simulink model "E55_1030"  (R2019b)
settings: Solver=FixedStepDiscrete  StartTime=0.0  StopTime=10  FixedStep=0.0005  RelTol=1e-3  EnableMultiTasking=on
InitFcn:
  | ecucoder_canfd
  | load('DATA_Plimit.mat')
  | a=0.775;
  | b=0.775;
  | kf=-50000;
  | kr=-50000;
  | m=226+75;
  | Iz=100;
  | u=0.85;
  | g=9.8;
  | L=a+b;
  | xi=0.1;
  | r=0.226;
  | Lw=1.171;
  | Tm=21;
  | i=15.9;
  | Jw=0.504;
  | Pmax=20000;
  | mw=19.3;
  | mb=148.9+75;
  | hg=0.280;
model workspace (MAT data in the model file):
  Initial_Steer_Position = 0
values from neighbouring files (symbols this model uses):
  SOC = [2.5 5 7.5 10 20 30 40 50 60 70 80 90 ... (14 elements, 14x1)]    [DATA_Plimit.mat]
  SOC_Discharge = [2.04592350211 2.57821618825 3.10671863859 3.63118835861 4.15200192786 4.66837694959 5.18149950051 5.69046162564 6.19532286188 6.696400261 7.19347596839 7.68712157998 ... (473 elements, 1x473)]    [DATA_Plimit.mat]
  VOLTAGE = [459.1488 476.0844 485.9448 487.344 492.822 498.8016 503.382 509.1108 518.8128 531.2472 544.5132 558.4656 ... (14 elements, 14x1)]    [DATA_Plimit.mat]
undefined symbols (not defined in the file or in its folder): DiscIntNeverNeededParam, H, HALL10, HALL6, HALL7, HALL8, HALL9, HPWM1, HPWM3, I_AN05_5V, I_AN07_5V, I_AN08_5V, I_AN09_5V, I_AN10_5V, I_SW11_H, I_SW12_H, I_SW13_H, I_SW14_H, I_SW15_H, I_SW16_H, I_SW17_H, I_SW18_H, I_SW19_H, LS1A2, O_HS1A2, O_HS1A8
libraries: ec311lib x152, simulink x92, canmsglib x30, canfdmsglib x2
(part 3 of 6)

== system E55_1030/Function-Call Subsystem3 ==
  CAN0 0X111 BMS CAN发送 : Inport
  function : TriggerPort  TriggerType=function-call  VariantControl=Variant
  Add : Sum
  Constant : Constant
  If : If  IfExpression=u1 >= 10
  If Action Subsystem : Subsystem  TreatAsAtomicUnit=on
  Saturation : Saturate  UpperLimit=10  LowerLimit=0
  Unit Delay : UnitDelay  SampleTime=-1  HasFrameUpgradeWarning=on
  wires:
  Unit Delay/1 -> Add/2
  Add/1 -> Saturation/1, Unit Delay/1
  Constant/1 -> Add/1
  CAN0 0X111 BMS CAN发送/1 -> If Action Subsystem/1(CAN0 0x111 BMS CAN发送)
  Saturation/1 -> If/1
  If/1 -> If Action Subsystem/Action

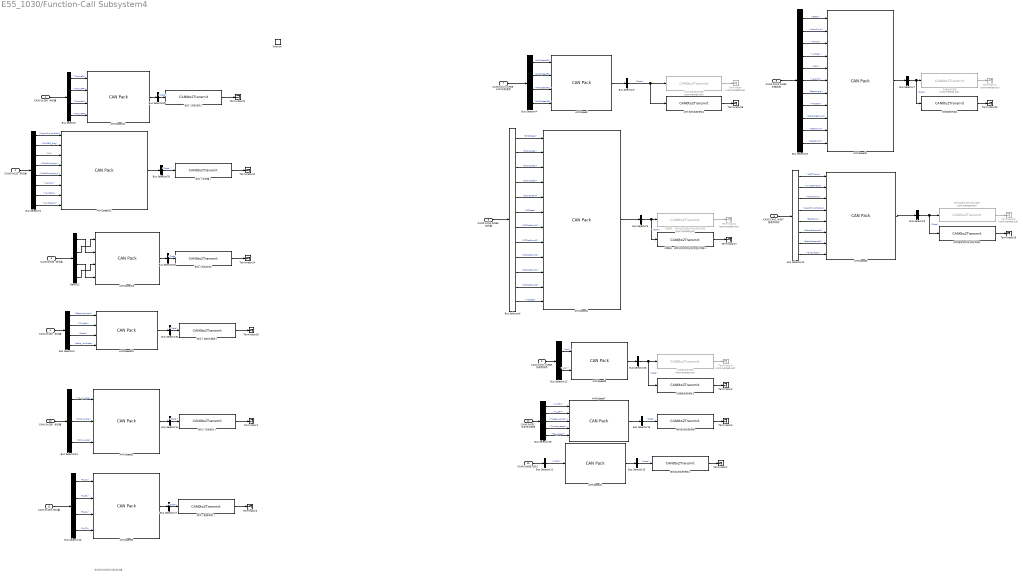
== system E55_1030/Function-Call Subsystem4 ==
  note: 驱动防滑和扭矩分配测试量
  CAN0 0x190 测试量 : Inport
  CAN0 0x191 测试量 : Inport  Port=2
  CAN0 0x192 测试量 : Inport  Port=3
  CAN0 0x194 测试量 : Inport  Port=4
  CAN0 CAN1 0x556 各种量 : Inport  Port=5
  CAN0 CAN1 0x557 温度和油压 : Inport  Port=6
  CAN0 CAN1 0x558 AMK电机速度 : Inport  Port=7
  CAN0 CAN1 0x559 车辆信息 : Inport  Port=8
  CAN0 CAN1 0x55B 加速度信息 : Inport  Port=9
  CAN0 0x195 测试量 : Inport  Port=10
  CAN0 0x193 测试量 : Inport  Port=11
  CAN0 0x55C 电机电流信息 : Inport  Port=12
  CAN0 0x55E vSOC : Inport  Port=13
  function : TriggerPort  TriggerType=function-call  VariantControl=Variant
  AMKSpeed : canmsglib/CAN Pack  MsgList=(none)  MsgName=AMKSpeed  MsgIDType=Standard (11-bit identifier)  MsgIdentifier=1368  MsgLength=8  Remote=off  ApplyMinMax=off  BusOutput=on  SignalInfo={ 'AMKSpeed1', '48', '16', 'LE', 'unsigned', 'Standard', '0', '1', '0', '0', '20000'; 'AMKSpeed2', '32', '16', 'LE', 'unsigned', 'Standard', '0', '1', '0', '0', '20000'; 'AMKSpeed3', '16', '16', 'LE', 'unsigned', 'Standard', '0', '1', '0', '0', '20000'; 'AMKSpeed4', '0', '16', 'LE', 'unsigned', 'Standard', '0', '1', '0', '0', '20000' }
      settings: SourceProductName=Vehicle Network Toolbox  SourceProductBaseCode=VN  DataFormat=manually specified signals
  AMKSpeed1 : canmsglib/CAN Pack  MsgList=(none)  MsgName=ErrorCode_State_Voltage  MsgIDType=Standard (11-bit identifier)  MsgIdentifier=1366  MsgLength=8  Remote=off  ApplyMinMax=off  BusOutput=on  SignalInfo={ 'BMS_State', '48', '1', 'LE', 'unsigned', 'Standard', '0', '1', '0', '0', '1'; 'Motor1_ErrorCode', '36', '12', 'LE', 'unsigned', 'Standard', '0', '1', '0', '0', '3871'; 'Motor2_ErrorCode', '24', '12', 'LE', 'unsigned', 'Standard', '0', '1', '0', '0', '3871'; 'Motor3_ErrorCode', '12', '12', 'LE', 'unsigned', 'Standard', '0', '1', '0', '0', '3871'; 'Motor4_ErrorCode', '0', '12', 'LE', 'unsigned', 'Standard', '0', '1', '0', '0', '3871'; 'SC_State', '49', '1', 'LE', 'unsigned', 'Standard', '0', '1', '0', '0', '1'; 'SC_TestPoint1', '50', '1', 'LE', 'unsigned', 'Standard', '0', '1', '0', '0', '1'; 'SC_TestPoint2', '51', '1', 'LE', 'unsigned', 'Standard', '0', '1', '0', '0', '1'; 'SC_TestPoint3', '52', '1', 'LE', 'unsigned', 'Standard', '0', '1', '0', '0', '1'; 'SC_TestPoint4', '53', '1', 'LE', 'unsigned', 'Standard', '0', '1', '0', '0', '1'; 'SC_TestPoint5', '54', '1', 'LE', 'unsigned', 'Standard', '0', '1', '0', '0', '1'; 'Voltage', '55', '9', 'LE', 'unsigned', 'Standard', '0', '0.1', '0', '0', '26' }
      settings: SourceProductName=Vehicle Network Toolbox  SourceProductBaseCode=VN  DataFormat=manually specified signals
  AMKSpeed11 : canmsglib/CAN Pack  MsgList=(none)  MsgName=Torque  MsgIDType=Standard (11-bit identifier)  MsgIdentifier=400  MsgLength=8  Remote=off  ApplyMinMax=off  BusOutput=on  SignalInfo={ 'TorqueFL', '16', '16', 'LE', 'signed', 'Standard', '0', '1', '0', '-Inf', 'Inf'; 'TorqueFR', '0', '16', 'LE', 'signed', 'Standard', '0', '1', '0', '-Inf', 'Inf'; 'TorqueRL', '48', '16', 'LE', 'signed', 'Standard', '0', '1', '0', '-Inf', 'Inf'; 'TorqueRR', '32', '16', 'LE', 'signed', 'Standard', '0', '1', '0', '-Inf', 'Inf' }
      settings: SourceProductName=Vehicle Network Toolbox  SourceProductBaseCode=VN  DataFormat=manually specified signals
  AMKSpeed12 : canmsglib/CAN Pack  MsgList=(none)  MsgName=Angle_Rate_Mz_Veloccity  MsgIDType=Standard (11-bit identifier)  MsgIdentifier=401  MsgLength=8  Remote=off  ApplyMinMax=off  BusOutput=on  SignalInfo={ 'Algorithm_Enable', '15', '1', 'LE', 'unsigned', 'Standard', '0', '1', '0', '0', '1'; 'K3105GStatus', '14', '1', 'LE', 'unsigned', 'Standard', '0', '1', '0', '0', '1'; 'Mz', '0', '14', 'LE', 'signed', 'Standard', '0', '0.05', '0', '-300', '300'; 'SideSlipAngle', '32', '8', 'LE', 'signed', 'Standard', '0', '0.1', '0', '-12.8', '12.7'; 'SideSlipAngle_d', '40', '8', 'LE', 'signed', 'Standard', '0', '0.1', '0', '-12.8', '12.7'; 'Velocity', '16', '16', 'LE', 'unsigned', 'Standard', '0', '0.01', '0', '0', '120'; 'YawRate', '48', '8', 'LE', 'signed', 'Standard', '0', '1', '0', '-128', '127'; 'YawRate_d', '56', '8', 'LE', 'signed', 'Standard', '0', '1', '0', '-128', '127' }
      settings: SourceProductName=Vehicle Network Toolbox  SourceProductBaseCode=VN  DataFormat=manually specified signals
  AMKSpeed13 : canmsglib/CAN Pack  MsgList=(none)  MsgName=Wheel_Speed  MsgIDType=Standard (11-bit identifier)  MsgIdentifier=402  MsgLength=8  Remote=off  ApplyMinMax=off  BusOutput=on  SignalInfo={ 'Wheel_Speed_FL', '0', '16', 'LE', 'signed', 'Standard', '0', '1', '0', '-1500', '1500'; 'Wheel_Speed_FR', '16', '16', 'LE', 'signed', 'Standard', '0', '1', '0', '-1500', '1500'; 'Wheel_Speed_RL', '32', '16', 'LE', 'signed', 'Standard', '0', '1', '0', '-1500', '1500'; 'Wheel_Speed_RR', '48', '16', 'LE', 'signed', 'Standard', '0', '1', '0', '-1500', '1500' }
      settings: SourceProductName=Vehicle Network Toolbox  SourceProductBaseCode=VN  DataFormat=manually specified signals
  AMKSpeed15 : canmsglib/CAN Pack  MsgList=(none)  MsgName=DriverIntention  MsgIDType=Standard (11-bit identifier)  MsgIdentifier=404  MsgLength=8  Remote=off  ApplyMinMax=off  BusOutput=on  SignalInfo={ 'SteeringAngle', '0', '12', 'LE', 'signed', 'Standard', '0', '0.01', '0', '-20', '20'; 'Throttle', '56', '8', 'LE', 'unsigned', 'Standard', '0', '1', '0', '0', '100'; 'break', '48', '8', 'LE', 'unsigned', 'Standard', '0', '1', '0', '0', '100'; 'delta_YawRate', '24', '8', 'LE', 'signed', 'Standard', '0', '1', '0', '-128', '127' }
      settings: SourceProductName=Vehicle Network Toolbox  SourceProductBaseCode=VN  DataFormat=manually specified signals
  AMKSpeed2 : canmsglib/CAN Pack  MsgList=(none)  MsgName=CarData  MsgIDType=Standard (11-bit identifier)  MsgIdentifier=1369  MsgLength=8  Remote=off  ApplyMinMax=off  BusOutput=on  SignalInfo={ 'Break', '51', '10', 'LE', 'unsigned', 'Standard', '0', '0.1', '0', '0', '100'; 'MotorAlive', '2', '4', 'LE', 'unsigned', 'Standard', '0', '1', '0', '0', '15'; 'Power', '17', '7', 'LE', 'signed', 'Standard', '0', '1', '44', '-20', '107'; 'RUN_Flag', '0', '2', 'LE', 'unsigned', 'Standard', '0', '1', '1', '1', '3'; 'SOC', '31', '10', 'LE', 'unsigned', 'Standard', '0', '0.1', '0', '0', '100'; 'Speed', '24', '7', 'LE', 'unsigned', 'Standard', '0', '1', '0', '0', '100'; 'SteerAngle', '6', '11', 'LE', 'signed', 'Standard', '0', '0.1', '0', '-100', '100'; 'Throttle', '41', '10', 'LE', 'unsigned', 'Standard', '0', '0.1', '0', '0', '100'; 'precharge_button', '63', '1', 'LE', 'unsigned', 'Standard', '0', '1', '0', '0', '1'; 'ready2go_button', '62', '1', 'LE', 'unsigned', 'Standard', '0', '1', '0', '0', '1'; 'reset_button', '61', '1', 'LE', 'unsigned', 'Standard', '0', '1', '0', '0', '1' }
      settings: SourceProductName=Vehicle Network Toolbox  SourceProductBaseCode=VN  DataFormat=manually specified signals
  AMKSpeed3 : canmsglib/CAN Pack  MsgList=(none)  MsgName=Temp_BreakPressure  MsgIDType=Standard (11-bit identifier)  MsgIdentifier=1367  MsgLength=8  Remote=off  ApplyMinMax=off  BusOutput=on  SignalInfo={ 'AMK_Temp_IGBT', '11', '11', 'LE', 'unsigned', 'Standard', '0', '0.1', '0', '0', '120'; 'AMK_Temp_Inverter', '22', '11', 'LE', 'unsigned', 'Standard', '0', '0.1', '0', '0', '120'; 'AMK_Temp_Motor', '33', '11', 'LE', 'unsigned', 'Standard', '0', '0.1', '0', '0', '120'; 'Algorithm_Enable', '63', '1', 'LE', 'unsigned', 'Standard', '0', '1', '0', '0', '1'; 'BattTemp', '0', '11', 'LE', 'unsigned', 'Standard', '0', '0.1', '0', '0', '120'; 'BreakPressure_F', '44', '9', 'LE', 'unsigned', 'Standard', '0', '0.05', '0', '0', '10'; 'BreakPressure_R', '53', '9', 'LE', 'unsigned', 'Standard', '0', '0.05', '0', '0', '10'; 'One_Motor', '62', '1', 'LE', 'unsigned', 'Standard', '0', '1', '0', '0', '1' }
      settings: SourceProductName=Vehicle Network Toolbox  SourceProductBaseCode=VN  DataFormat=manually specified signals
  AMKSpeed4 : canmsglib/CAN Pack  MsgList=(none)  MsgName=Dashboard_Control  MsgIDType=Standard (11-bit identifier)  MsgIdentifier=1374  MsgLength=8  Remote=off  ApplyMinMax=off  BusOutput=on  SignalInfo={ 'vSOC', '8', '16', 'LE', 'unsigned', 'Standard', '0', '0.01', '0', '0', '100' }
      settings: SourceProductName=Vehicle Network Toolbox  SourceProductBaseCode=VN  DataFormat=manually specified signals
  AMKSpeed5 : canmsglib/CAN Pack  MsgList=(none)  MsgName=Attitude  MsgIDType=Standard (11-bit identifier)  MsgIdentifier=405  MsgLength=8  Remote=off  ApplyMinMax=off  BusOutput=on  SignalInfo={ 'Heading_Angle', '0', '16', 'LE', 'unsigned', 'Standard', '0', '0.01', '0', '0', '360'; 'Pitch_Angle', '24', '16', 'LE', 'signed', 'Standard', '0', '0.01', '0', '-180', '180'; 'Roll_Angle', '48', '16', 'LE', 'signed', 'Standard', '0', '0.01', '0', '-180', '180' }
      settings: SourceProductName=Vehicle Network Toolbox  SourceProductBaseCode=VN  DataFormat=manually specified signals
  AMKSpeed6 : canmsglib/CAN Pack  MsgList=(none)  MsgName=Fz  MsgIDType=Standard (11-bit identifier)  MsgIdentifier=403  MsgLength=8  Remote=off  ApplyMinMax=off  BusOutput=on  SignalInfo={ 'Fz_FL', '0', '16', 'LE', 'unsigned', 'Standard', '0', '0.05', '0', '0', '2000'; 'Fz_FR', '16', '16', 'LE', 'unsigned', 'Standard', '0', '0.05', '0', '0', '2000'; 'Fz_RL', '32', '16', 'LE', 'unsigned', 'Standard', '0', '0.05', '0', '0', '2000'; 'Fz_RR', '48', '16', 'LE', 'unsigned', 'Standard', '0', '0.05', '0', '0', '2000' }
      settings: SourceProductName=Vehicle Network Toolbox  SourceProductBaseCode=VN  DataFormat=manually specified signals
  AMKSpeed7 : canmsglib/CAN Pack  MsgList=(none)  MsgName=Current  MsgIDType=Standard (11-bit identifier)  MsgIdentifier=1372  MsgLength=8  Remote=off  ApplyMinMax=off  BusOutput=on  SignalInfo={ 'Id_284', '0', '16', 'LE', 'signed', 'Standard', '0', '0.001', '0', '-10', '20'; 'Iq_284', '16', '16', 'LE', 'signed', 'Standard', '0', '0.001', '0', '-10', '20'; 'Target_velocity', '32', '16', 'LE', 'signed', 'Standard', '0', '1', '0', '-5000', '20000'; 'Torque_regen', '49', '15', 'LE', 'signed', 'Standard', '0', '0.1', '0', '-1000', '0'; 'flag_regen', '48', '1', 'LE', 'unsigned', 'Standard', '0', '1', '0', '0', '1' }
      settings: SourceProductName=Vehicle Network Toolbox  SourceProductBaseCode=VN  DataFormat=manually specified signals
  AMKSpeed9 : canmsglib/CAN Pack  MsgList=(none)  MsgName=Acceleration  MsgIDType=Standard (11-bit identifier)  MsgIdentifier=1371  MsgLength=8  Remote=off  ApplyMinMax=off  BusOutput=on  SignalInfo={ 'Acceleration_X', '0', '16', 'LE', 'signed', 'Standard', '0', '0.01', '0', '-40', '40'; 'Acceleration_Y', '16', '16', 'LE', 'signed', 'Standard', '0', '0.01', '0', '-40', '40' }
      settings: SourceProductName=Vehicle Network Toolbox  SourceProductBaseCode=VN  DataFormat=manually specified signals
  AMK电机速度传输 : ec311lib/RapidECU_U34/03CANCommunication/CAN0to2Transmit  Commented=on  canmodule=1  canbuffer=29  canmessageid=hex2dec('0558')  canmessagetype=Standard(11-bit ID)  datalength=8  sampletime=-1
      settings: SourceProductName=ECUCoder for S32K311
  AMK电机速度传输1 : ec311lib/RapidECU_U34/03CANCommunication/CAN0to2Transmit  canmodule=0  canbuffer=29  canmessageid=hex2dec('0558')  canmessagetype=Standard(11-bit ID)  datalength=8  sampletime=-1
      settings: SourceProductName=ECUCoder for S32K311
  Bus Selector : BusSelector  OutputSignals=TorqueFL,TorqueFR,TorqueRL,TorqueRR
  Bus Selector1 : BusSelector  OutputSignals=Algorithm_Enable,K3105G_flag,Mz,SideSlipAngle,SideSlipAngle_d,velocity,YawRate,YawRate_d
  Bus Selector10 : BusSelector  OutputSignals=IGBTTemp,InverterTemp,MotorTemp,Algorithm_Enable,BattTemp,BreakPressureF,BreakPressureR,One_Motor
  Bus Selector11 : BusSelector  OutputSignals=vSOC
  Bus Selector12 : BusSelector  OutputSignals=AccX,AccY
  Bus Selector13 : BusSelector  OutputSignals=Yaw_Angle,Pitch_Angle,Roll_Angle
  Bus Selector{3,5,7,9,14..15,17..18,26,28..30,32} (13 alike) : BusSelector  OutputSignals=Data
  Bus Selector16 : BusSelector  OutputSignals=Fz_FL,Fz_FR,Fz_RL,Fz_RR
  Bus Selector19 : BusSelector  OutputSignals=Id_284,Iq_284,Target_velocity,Torque_regen,flag_regen
  Bus Selector2 : BusSelector  OutputSignals=SteeringAngle,Throttle,Break,delta_YawRate
  Bus Selector4 : BusSelector  OutputSignals=AMKSpeedFL,AMKSpeedFR,AMKSpeedRL,AMKSpeedRR
  Bus Selector6 : BusSelector  OutputSignals=BMSState,ErrorCode1,ErrorCode2,ErrorCode3,ErrorCode4,SCState,SCTestPoint1,SCTestPoint2,SCTestPoint3,SCTestPoint4,SCTestPoint5,Voltage
  Bus Selector8 : BusSelector  OutputSignals=Break,MotorAlive,Power,runflag,SOC,velocity,SteerAngle,Throttle,PrechargeInput,StartInput,ResetInput
  Demux2 : Demux
  Terminator{,4,7..9} (5 alike) : Terminator  Commented=on
  Terminator{1..3,5..6,22,24..28,30..31} (13 alike) : Terminator
  加速度信息传输 : ec311lib/RapidECU_U34/03CANCommunication/CAN0to2Transmit  Commented=on  canmodule=1  canbuffer=1  canmessageid=hex2dec('055B')  canmessagetype=Standard(11-bit ID)  datalength=8  sampletime=-1
      settings: SourceProductName=ECUCoder for S32K311
  加速度信息传输1 : ec311lib/RapidECU_U34/03CANCommunication/CAN0to2Transmit  canmodule=0  canbuffer=1  canmessageid=hex2dec('055B')  canmessagetype=Standard(11-bit ID)  datalength=8  sampletime=-1
      settings: SourceProductName=ECUCoder for S32K311
  各种温度和刹车油压传输 : ec311lib/RapidECU_U34/03CANCommunication/CAN0to2Transmit  Commented=on  canmodule=1  canbuffer=31  canmessageid=hex2dec('0557')  canmessagetype=Standard(11-bit ID)  datalength=8  sampletime=-1
      settings: SourceProductName=ECUCoder for S32K311
  各种温度和刹车油压传输1 : ec311lib/RapidECU_U34/03CANCommunication/CAN0to2Transmit  canmodule=0  canbuffer=31  canmessageid=hex2dec('0557')  canmessagetype=Standard(11-bit ID)  datalength=8  sampletime=-1
      settings: SourceProductName=ECUCoder for S32K311
  故障码、各种状态和低压电池电压传输 : ec311lib/RapidECU_U34/03CANCommunication/CAN0to2Transmit  Commented=on  canmodule=1  canbuffer=30  canmessageid=hex2dec('0556')  canmessagetype=Standard(11-bit ID)  datalength=8  sampletime=-1
      settings: SourceProductName=ECUCoder for S32K311
  故障码、各种状态和低压电池电压传输1 : ec311lib/RapidECU_U34/03CANCommunication/CAN0to2Transmit  canmodule=0  canbuffer=30  canmessageid=hex2dec('0556')  canmessagetype=Standard(11-bit ID)  datalength=8  sampletime=-1
      settings: SourceProductName=ECUCoder for S32K311
  测试（各种量） : ec311lib/RapidECU_U34/03CANCommunication/CAN0to2Transmit  canmodule=0  canbuffer=13  canmessageid=hex2dec('0191')  canmessagetype=Standard(11-bit ID)  datalength=8  sampletime=-1
      settings: SourceProductName=ECUCoder for S32K311
  测试（四轮扭矩） : ec311lib/RapidECU_U34/03CANCommunication/CAN0to2Transmit  canmodule=0  canbuffer=12  canmessageid=hex2dec('0190')  canmessagetype=Standard(11-bit ID)  datalength=8  sampletime=-1
      settings: SourceProductName=ECUCoder for S32K311
  测试（四轮轮速） : ec311lib/RapidECU_U34/03CANCommunication/CAN0to2Transmit  canmodule=0  canbuffer=14  canmessageid=hex2dec('0192')  canmessagetype=Standard(11-bit ID)  datalength=8  sampletime=-1
      settings: SourceProductName=ECUCoder for S32K311
  测试（垂直载荷） : ec311lib/RapidECU_U34/03CANCommunication/CAN0to2Transmit  canmodule=0  canbuffer=17  canmessageid=hex2dec('0193')  canmessagetype=Standard(11-bit ID)  datalength=8  sampletime=-1
      settings: SourceProductName=ECUCoder for S32K311
  测试（车身姿态） : ec311lib/RapidECU_U34/03CANCommunication/CAN0to2Transmit  canmodule=0  canbuffer=18  canmessageid=hex2dec('0195')  canmessagetype=Standard(11-bit ID)  datalength=8  sampletime=-1
      settings: SourceProductName=ECUCoder for S32K311
  测试（驾驶员意图） : ec311lib/RapidECU_U34/03CANCommunication/CAN0to2Transmit  canmodule=0  canbuffer=16  canmessageid=hex2dec('0194')  canmessagetype=Standard(11-bit ID)  datalength=8  sampletime=-1
      settings: SourceProductName=ECUCoder for S32K311
  电机电流信息传输 : ec311lib/RapidECU_U34/03CANCommunication/CAN0to2Transmit  canmodule=0  canbuffer=33  canmessageid=hex2dec('055C')  canmessagetype=Standard(11-bit ID)  datalength=8  sampletime=-1
      settings: SourceProductName=ECUCoder for S32K311
  电机电流信息传输1 : ec311lib/RapidECU_U34/03CANCommunication/CAN0to2Transmit  canmodule=0  canbuffer=34  canmessageid=hex2dec('055E')  canmessagetype=Standard(11-bit ID)  datalength=8  sampletime=-1
      settings: SourceProductName=ECUCoder for S32K311
  车辆信息传输 : ec311lib/RapidECU_U34/03CANCommunication/CAN0to2Transmit  Commented=on  canmodule=1  canbuffer=32  canmessageid=hex2dec('0559')  canmessagetype=Standard(11-bit ID)  datalength=8  sampletime=-1
      settings: SourceProductName=ECUCoder for S32K311
  车辆信息传输1 : ec311lib/RapidECU_U34/03CANCommunication/CAN0to2Transmit  canmodule=0  canbuffer=32  canmessageid=hex2dec('0559')  canmessagetype=Standard(11-bit ID)  datalength=8  sampletime=-1
      settings: SourceProductName=ECUCoder for S32K311
  wires:
  测试（四轮扭矩）/1 -> Terminator31/1
  测试（驾驶员意图）/1 -> Terminator30/1
  测试（各种量）/1 -> Terminator22/1
  测试（四轮轮速）/1 -> Terminator24/1
  车辆信息传输1/1 -> Terminator25/1
  各种温度和刹车油压传输1/1 -> Terminator26/1
  各种温度和刹车油压传输/1 -> Terminator8/1
  车辆信息传输/1 -> Terminator7/1
  故障码、各种状态和低压电池电压传输/1 -> Terminator4/1
  故障码、各种状态和低压电池电压传输1/1 -> Terminator27/1
  AMK电机速度传输/1 -> Terminator/1
  AMK电机速度传输1/1 -> Terminator28/1
  加速度信息传输/1 -> Terminator9/1
  AMKSpeed11/1 -> Bus Selector29/1
  Bus Selector29/1 -> 测试（四轮扭矩）/1  "<Data>"
  CAN0 0x190 测试量/1 -> Bus Selector/1
  Bus Selector/1 -> AMKSpeed11/1  "<TorqueFL>"
  Bus Selector/2 -> AMKSpeed11/2  "<TorqueFR>"
  Bus Selector/3 -> AMKSpeed11/3  "<TorqueRL>"
  Bus Selector/4 -> AMKSpeed11/4  "<TorqueRR>"
  AMKSpeed12/1 -> Bus Selector28/1
  Bus Selector28/1 -> 测试（各种量）/1  "<Data>"
  CAN0 0x191 测试量/1 -> Bus Selector1/1
  Demux2/1 -> AMKSpeed13/2
  Demux2/3 -> AMKSpeed13/4
  Demux2/2 -> AMKSpeed13/1
  Demux2/4 -> AMKSpeed13/3
  AMKSpeed13/1 -> Bus Selector30/1
  CAN0 0x192 测试量/1 -> Demux2/1
  Bus Selector30/1 -> 测试（四轮轮速）/1  "<Data>"
  AMKSpeed15/1 -> Bus Selector32/1
  Bus Selector32/1 -> 测试（驾驶员意图）/1  "<Data>"
  CAN0 0x194 测试量/1 -> Bus Selector2/1
  AMKSpeed/1 -> Bus Selector3/1
  CAN0 CAN1 0x558 AMK电机速度/1 -> Bus Selector4/1
  Bus Selector4/1 -> AMKSpeed/1  "<AMKSpeedFL>"
  Bus Selector4/2 -> AMKSpeed/2  "<AMKSpeedFR>"
  Bus Selector4/3 -> AMKSpeed/3  "<AMKSpeedRL>"
  Bus Selector4/4 -> AMKSpeed/4  "<AMKSpeedRR>"
  Bus Selector3/1 -> AMK电机速度传输1/1, AMK电机速度传输/1  "<Data>"
  AMKSpeed1/1 -> Bus Selector5/1
  Bus Selector5/1 -> 故障码、各种状态和低压电池电压传输1/1, 故障码、各种状态和低压电池电压传输/1  "<Data>"
  CAN0 CAN1 0x556 各种量/1 -> Bus Selector6/1
  Bus Selector6/1 -> AMKSpeed1/1  "<BMSState>"
  Bus Selector6/2 -> AMKSpeed1/2  "<ErrorCode1>"
  Bus Selector6/3 -> AMKSpeed1/3  "<ErrorCode2>"
  Bus Selector6/4 -> AMKSpeed1/4  "<ErrorCode3>"
  Bus Selector6/5 -> AMKSpeed1/5  "<ErrorCode4>"
  Bus Selector6/6 -> AMKSpeed1/6  "<SCState>"
  Bus Selector6/7 -> AMKSpeed1/7  "<SCTestPoint1>"
  Bus Selector6/8 -> AMKSpeed1/8  "<SCTestPoint2>"
  Bus Selector6/9 -> AMKSpeed1/9  "<SCTestPoint3>"
  Bus Selector6/10 -> AMKSpeed1/10  "<SCTestPoint4>"
  Bus Selector6/11 -> AMKSpeed1/11  "<SCTestPoint5>"
  Bus Selector6/12 -> AMKSpeed1/12  "<Voltage>"
  AMKSpeed2/1 -> Bus Selector7/1
  Bus Selector7/1 -> 车辆信息传输1/1, 车辆信息传输/1  "<Data>"
  CAN0 CAN1 0x559 车辆信息/1 -> Bus Selector8/1
  Bus Selector8/1 -> AMKSpeed2/1  "<Break>"
  Bus Selector8/2 -> AMKSpeed2/2  "<MotorAlive>"
  Bus Selector8/3 -> AMKSpeed2/3  "<Power>"
  Bus Selector8/4 -> AMKSpeed2/4  "<runflag>"
  Bus Selector8/5 -> AMKSpeed2/5  "<SOC>"
  Bus Selector8/6 -> AMKSpeed2/6  "<velocity>"
  Bus Selector8/7 -> AMKSpeed2/7  "<SteerAngle>"
  Bus Selector8/8 -> AMKSpeed2/8  "<Throttle>"
  Bus Selector8/9 -> AMKSpeed2/9  "<PrechargeInput>"
  Bus Selector8/10 -> AMKSpeed2/10  "<StartInput>"
  Bus Selector8/11 -> AMKSpeed2/11  "<ResetInput>"
  AMKSpeed3/1 -> Bus Selector9/1
  Bus Selector9/1 -> 各种温度和刹车油压传输1/1, 各种温度和刹车油压传输/1  "<Data>"
  CAN0 CAN1 0x557 温度和油压/1 -> Bus Selector10/1
  Bus Selector10/1 -> AMKSpeed3/1  "<IGBTTemp>"
  Bus Selector10/2 -> AMKSpeed3/2  "<InverterTemp>"
  Bus Selector10/3 -> AMKSpeed3/3  "<MotorTemp>"
  AMKSpeed9/1 -> Bus Selector26/1
  Bus Selector26/1 -> 加速度信息传输1/1, 加速度信息传输/1  "<Data>"
  CAN0 CAN1 0x55B 加速度信息/1 -> Bus Selector12/1
  Bus Selector12/1 -> AMKSpeed9/1  "<AccX>"
  Bus Selector12/2 -> AMKSpeed9/2  "<AccY>"
  Bus Selector10/5 -> AMKSpeed3/5  "<BattTemp>"
  Bus Selector10/6 -> AMKSpeed3/6  "<BreakPressureF>"
  Bus Selector10/7 -> AMKSpeed3/7  "<BreakPressureR>"
  Bus Selector10/4 -> AMKSpeed3/4  "<Algorithm_Enable>"
  Bus Selector1/1 -> AMKSpeed12/1  "<Algorithm_Enable>"
  Bus Selector1/2 -> AMKSpeed12/2  "<K3105G_flag>"
  Bus Selector1/3 -> AMKSpeed12/3  "<Mz>"
  Bus Selector1/4 -> AMKSpeed12/4  "<SideSlipAngle>"
  Bus Selector1/5 -> AMKSpeed12/5  "<SideSlipAngle_d>"
  Bus Selector1/6 -> AMKSpeed12/6  "<velocity>"
  Bus Selector1/7 -> AMKSpeed12/7  "<YawRate>"
  Bus Selector1/8 -> AMKSpeed12/8  "<YawRate_d>"
  Bus Selector14/1 -> 测试（车身姿态）/1  "<Data>"
  CAN0 0x195 测试量/1 -> Bus Selector13/1
  测试（车身姿态）/1 -> Terminator1/1
  AMKSpeed5/1 -> Bus Selector14/1
  Bus Selector13/1 -> AMKSpeed5/1  "<Yaw_Angle>"
  Bus Selector13/2 -> AMKSpeed5/2  "<Pitch_Angle>"
  Bus Selector13/3 -> AMKSpeed5/3  "<Roll_Angle>"
  加速度信息传输1/1 -> Terminator3/1
  Bus Selector2/1 -> AMKSpeed15/1  "<SteeringAngle>"
  Bus Selector2/2 -> AMKSpeed15/2  "<Throttle>"
  Bus Selector2/3 -> AMKSpeed15/3  "<Break>"
  Bus Selector10/8 -> AMKSpeed3/8  "<One_Motor>"
  Bus Selector2/4 -> AMKSpeed15/4  "<delta_YawRate>"
  AMKSpeed6/1 -> Bus Selector17/1
  测试（垂直载荷）/1 -> Terminator5/1
  Bus Selector17/1 -> 测试（垂直载荷）/1  "<Data>"
  CAN0 0x193 测试量/1 -> Bus Selector16/1
  Bus Selector16/4 -> AMKSpeed6/4  "<Fz_RR>"
  Bus Selector16/3 -> AMKSpeed6/3  "<Fz_RL>"
  Bus Selector16/2 -> AMKSpeed6/2  "<Fz_FR>"
  Bus Selector16/1 -> AMKSpeed6/1  "<Fz_FL>"
  AMKSpeed7/1 -> Bus Selector18/1
  Bus Selector18/1 -> 电机电流信息传输/1  "<Data>"
  电机电流信息传输/1 -> Terminator6/1
  CAN0 0x55C 电机电流信息/1 -> Bus Selector19/1
  Bus Selector19/1 -> AMKSpeed7/1  "<Id_284>"
  Bus Selector19/2 -> AMKSpeed7/2  "<Iq_284>"
  Bus Selector19/4 -> AMKSpeed7/4  "<Torque_regen>"
  Bus Selector19/5 -> AMKSpeed7/5  "<flag_regen>"
  Bus Selector19/3 -> AMKSpeed7/3  "<Target_velocity>"
  CAN0 0x55E vSOC/1 -> Bus Selector11/1
  Bus Selector11/1 -> AMKSpeed4/1  "<vSOC>"
  电机电流信息传输1/1 -> Terminator2/1
  Bus Selector15/1 -> 电机电流信息传输1/1  "<Data>"
  AMKSpeed4/1 -> Bus Selector15/1

== system E55_1030/Function-Call Subsystem5 ==
  CAN2 0x185 右前 : Inport
  CAN2 0x184 左前 : Inport  Port=2
  CAN2 0x189 右后 : Inport  Port=3
  CAN2 0x188 左后 : Inport  Port=4
  function : TriggerPort  TriggerType=function-call  VariantControl=Variant
  AMKSpeed5 : canmsglib/CAN Pack  MsgList=(none)  MsgName=VCU4_0x184  MsgIDType=Standard (11-bit identifier)  MsgIdentifier=388  MsgLength=8  Remote=off  ApplyMinMax=off  BusOutput=on  SignalInfo={ 'DcOn', '9', '1', 'LE', 'unsigned', 'Standard', '0', '1', '0', '0', '1'; 'Enable', '10', '1', 'LE', 'unsigned', 'Standard', '0', '1', '0', '0', '1'; 'ErrorReset', '11', '1', 'LE', 'unsigned', 'Standard', '0', '1', '0', '0', '1'; 'InverterOn', '8', '1', 'LE', 'unsigned', 'Standard', '0', '1', '0', '-Inf', 'Inf'; 'TargetVelocity', '16', '16', 'LE', 'signed', 'Standard', '0', '1', '0', '-32768', '32767'; 'TorqueLimitNegativ', '48', '16', 'LE', 'signed', 'Standard', '0', '1', '0', '-32768', '32767'; 'TorqueLimitPositiv', '32', '16', 'LE', 'signed', 'Standard', '0', '1', '0', '-32768', '32767' }
      settings: SourceProductName=Vehicle Network Toolbox  SourceProductBaseCode=VN  DataFormat=manually specified signals
  AMKSpeed6 : canmsglib/CAN Pack  MsgList=(none)  MsgName=VCU4_0x185  MsgIDType=Standard (11-bit identifier)  MsgIdentifier=389  MsgLength=8  Remote=off  ApplyMinMax=off  BusOutput=on  SignalInfo={ 'DcOn', '9', '1', 'LE', 'unsigned', 'Standard', '0', '1', '0', '0', '1'; 'Enable', '10', '1', 'LE', 'unsigned', 'Standard', '0', '1', '0', '0', '1'; 'ErrorReset', '11', '1', 'LE', 'unsigned', 'Standard', '0', '1', '0', '0', '1'; 'InverterOn', '8', '1', 'LE', 'unsigned', 'Standard', '0', '1', '0', '-Inf', 'Inf'; 'TargetVelocity', '16', '16', 'LE', 'signed', 'Standard', '0', '1', '0', '-32768', '32767'; 'TorqueLimitNegativ', '48', '16', 'LE', 'signed', 'Standard', '0', '1', '0', '-32768', '32767'; 'TorqueLimitPositiv', '32', '16', 'LE', 'signed', 'Standard', '0', '1', '0', '-32768', '32767' }
      settings: SourceProductName=Vehicle Network Toolbox  SourceProductBaseCode=VN  DataFormat=manually specified signals
  AMKSpeed7 : canmsglib/CAN Pack  MsgList=(none)  MsgName=VCU4_0x189  MsgIDType=Standard (11-bit identifier)  MsgIdentifier=393  MsgLength=8  Remote=off  ApplyMinMax=off  BusOutput=on  SignalInfo={ 'DcOn', '9', '1', 'LE', 'unsigned', 'Standard', '0', '1', '0', '0', '1'; 'Enable', '10', '1', 'LE', 'unsigned', 'Standard', '0', '1', '0', '0', '1'; 'ErrorReset', '11', '1', 'LE', 'unsigned', 'Standard', '0', '1', '0', '0', '1'; 'InverterOn', '8', '1', 'LE', 'unsigned', 'Standard', '0', '1', '0', '-Inf', 'Inf'; 'TargetVelocity', '16', '16', 'LE', 'signed', 'Standard', '0', '1', '0', '-Inf', 'Inf'; 'TorqueLimitNegativ', '48', '16', 'LE', 'signed', 'Standard', '0', '1', '0', '-Inf', 'Inf'; 'TorqueLimitPositiv', '32', '16', 'LE', 'signed', 'Standard', '0', '1', '0', '-Inf', 'Inf' }
      settings: SourceProductName=Vehicle Network Toolbox  SourceProductBaseCode=VN  DataFormat=manually specified signals
  AMKSpeed8 : canmsglib/CAN Pack  MsgList=(none)  MsgName=VCU4_0x188  MsgIDType=Standard (11-bit identifier)  MsgIdentifier=392  MsgLength=8  Remote=off  ApplyMinMax=off  BusOutput=on  SignalInfo={ 'DcOn', '9', '1', 'LE', 'unsigned', 'Standard', '0', '1', '0', '0', '1'; 'Enable', '10', '1', 'LE', 'unsigned', 'Standard', '0', '1', '0', '0', '1'; 'ErrorReset', '11', '1', 'LE', 'unsigned', 'Standard', '0', '1', '0', '0', '1'; 'InverterOn', '8', '1', 'LE', 'unsigned', 'Standard', '0', '1', '0', '-Inf', 'Inf'; 'TargetVelocity', '16', '16', 'LE', 'signed', 'Standard', '0', '1', '0', '-32768', '32767'; 'TorqueLimitNegativ', '48', '16', 'LE', 'signed', 'Standard', '0', '1', '0', '-32768', '32767'; 'TorqueLimitPositiv', '32', '16', 'LE', 'signed', 'Standard', '0', '1', '0', '-32768', '32767' }
      settings: SourceProductName=Vehicle Network Toolbox  SourceProductBaseCode=VN  DataFormat=manually specified signals
  Bus Selector{,1..3} (4 alike) : BusSelector  OutputSignals=DcOn,Enable,ErrorReset,InverterOn,TargetVelocity,NegTorque,PosTorque
  Bus Selector{19,21,23,25} (4 alike) : BusSelector  OutputSignals=Data
  Terminator{12..15} (4 alike) : Terminator
  右前 : ec311lib/RapidECU_U34/03CANCommunication/CAN0to2Transmit  canmodule=2  canbuffer=8  canmessageid=hex2dec('0185')  canmessagetype=Standard(11-bit ID)  datalength=8  sampletime=-1
      settings: SourceProductName=ECUCoder for S32K311
  右后 : ec311lib/RapidECU_U34/03CANCommunication/CAN0to2Transmit  canmodule=2  canbuffer=11  canmessageid=hex2dec('0189')  canmessagetype=Standard(11-bit ID)  datalength=8  sampletime=-1
      settings: SourceProductName=ECUCoder for S32K311
  左前 : ec311lib/RapidECU_U34/03CANCommunication/CAN0to2Transmit  canmodule=2  canbuffer=7  canmessageid=hex2dec('0184')  canmessagetype=Standard(11-bit ID)  datalength=8  sampletime=-1
      settings: SourceProductName=ECUCoder for S32K311
  左后 : ec311lib/RapidECU_U34/03CANCommunication/CAN0to2Transmit  canmodule=2  canbuffer=10  canmessageid=hex2dec('0188')  canmessagetype=Standard(11-bit ID)  datalength=8  sampletime=-1
      settings: SourceProductName=ECUCoder for S32K311
  wires:
  左后/1 -> Terminator15/1
  右后/1 -> Terminator14/1
  左前/1 -> Terminator13/1
  右前/1 -> Terminator12/1
  AMKSpeed6/1 -> Bus Selector19/1
  Bus Selector19/1 -> 右前/1  "<Data>"
  CAN2 0x185 右前/1 -> Bus Selector/1
  Bus Selector/1 -> AMKSpeed6/1  "<DcOn>"
  Bus Selector/5 -> AMKSpeed6/5  "<TargetVelocity>"
  Bus Selector/6 -> AMKSpeed6/6  "<NegTorque>"
  Bus Selector/7 -> AMKSpeed6/7  "<PosTorque>"
  Bus Selector/2 -> AMKSpeed6/2  "<Enable>"
  Bus Selector/3 -> AMKSpeed6/3  "<ErrorReset>"
  Bus Selector/4 -> AMKSpeed6/4  "<InverterOn>"
  AMKSpeed7/1 -> Bus Selector23/1
  Bus Selector23/1 -> 右后/1  "<Data>"
  CAN2 0x189 右后/1 -> Bus Selector1/1
  Bus Selector1/1 -> AMKSpeed7/1  "<DcOn>"
  Bus Selector1/2 -> AMKSpeed7/2  "<Enable>"
  Bus Selector1/3 -> AMKSpeed7/3  "<ErrorReset>"
  Bus Selector1/4 -> AMKSpeed7/4  "<InverterOn>"
  Bus Selector1/5 -> AMKSpeed7/5  "<TargetVelocity>"
  Bus Selector1/6 -> AMKSpeed7/6  "<NegTorque>"
  Bus Selector1/7 -> AMKSpeed7/7  "<PosTorque>"
  AMKSpeed5/1 -> Bus Selector21/1
  Bus Selector21/1 -> 左前/1  "<Data>"
  CAN2 0x184 左前/1 -> Bus Selector2/1
  Bus Selector2/1 -> AMKSpeed5/1  "<DcOn>"
  Bus Selector2/2 -> AMKSpeed5/2  "<Enable>"
  Bus Selector2/3 -> AMKSpeed5/3  "<ErrorReset>"
  Bus Selector2/4 -> AMKSpeed5/4  "<InverterOn>"
  Bus Selector2/5 -> AMKSpeed5/5  "<TargetVelocity>"
  Bus Selector2/6 -> AMKSpeed5/6  "<NegTorque>"
  Bus Selector2/7 -> AMKSpeed5/7  "<PosTorque>"
  AMKSpeed8/1 -> Bus Selector25/1
  Bus Selector25/1 -> 左后/1  "<Data>"
  CAN2 0x188 左后/1 -> Bus Selector3/1
  Bus Selector3/1 -> AMKSpeed8/1  "<DcOn>"
  Bus Selector3/2 -> AMKSpeed8/2  "<Enable>"
  Bus Selector3/3 -> AMKSpeed8/3  "<ErrorReset>"
  Bus Selector3/4 -> AMKSpeed8/4  "<InverterOn>"
  Bus Selector3/5 -> AMKSpeed8/5  "<TargetVelocity>"
  Bus Selector3/6 -> AMKSpeed8/6  "<NegTorque>"
  Bus Selector3/7 -> AMKSpeed8/7  "<PosTorque>"

== system E55_1030/Initializationl Subsystem ==
  function : TriggerPort  TriggerType=function-call  VariantControl=(inherit)
  MeaModule9 : ec311lib/RapidECU_U34/09Calibration/MeaModule  signal=LVBatteryVolt
      settings: SourceProductName=ECUCoder for S32K311
  PowerVoltageMonitor : ec311lib/RapidECU_U34/07PowerManagement/PowerVoltageMonitor  channel=4-5: I_BAT  sampletime=-1
      settings: SourceProductName=ECUCoder for S32K311
  Terminator : Terminator
  wires:
  PowerVoltageMonitor/1 -> MeaModule9/1
  MeaModule9/1 -> Terminator/1

== system E55_1030/Function-Call Subsystem2/Function-Call Subsystem ==
  CAN_OK : Inport
  "CAN_ID " : Inport  Port=2
  CAN_MSG : Inport  Port=3
  function : TriggerPort  TriggerType=function-call  VariantControl=Variant
  Bus Creator : BusCreator  Inputs=2
  Enabled Subsystem : Subsystem  TreatAsAtomicUnit=on
  Dashboard_Control : Outport
  wires:
  CAN_OK/1 -> Enabled Subsystem/Enable, Bus Creator/1  "CAN_OK"
  "CAN_ID "/1 -> Enabled Subsystem/1(CAN_ID)
  CAN_MSG/1 -> Enabled Subsystem/2(CAN_MSG)
  Enabled Subsystem/1(K3105_Alive) -> Bus Creator/2  "K3105_Alive"
  Bus Creator/1 -> Dashboard_Control/1

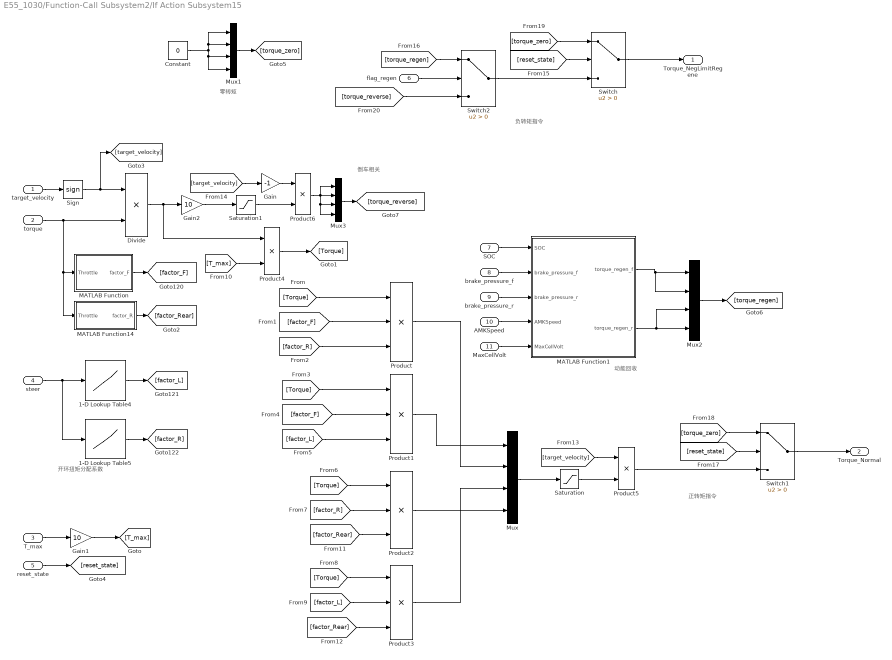
== system E55_1030/Function-Call Subsystem2/If Action Subsystem15 ==
  note: 倒车相关
  note: 开环扭矩分配系数
  note: 正转矩指令
  note: 动能回收
  note: 负转矩指令
  note: 零转矩
  target_velocity : Inport
  torque : Inport  Port=2
  T_max : Inport  Port=3
  steer : Inport  Port=4
  reset_state : Inport  Port=5
  flag_regen : Inport  Port=6
  SOC : Inport  Port=7
  brake_pressure_f : Inport  Port=8
  brake_pressure_r : Inport  Port=9
  AMKSpeed : Inport  Port=10
  MaxCellVolt : Inport  Port=11
  1-D Lookup Table4 : Lookup_n-D  NumberOfTableDimensions=1  BreakpointsForDimension1=[-110,-100,-60,-20,20,60,90,100]  Table=[1.5,1.5,1.3,1,1,0.8,0.5,0.5]  InternalRulePriority=Speed  RndMeth=Simplest  InputSameDT=on
  1-D Lookup Table5 : Lookup_n-D  NumberOfTableDimensions=1  BreakpointsForDimension1=[-110,-100,-60,-20,20,60,90,100]  Table=[0.5,0.5,0.8,1,1,1.3,1.5,1.5]  InternalRulePriority=Speed  RndMeth=Simplest  InputSameDT=on
  Constant : Constant  Value=0
  Divide : Product  Inputs=**
  Gain : Gain  Gain=-1
  Gain1 : Gain  Gain=10
  Gain2 : Gain  Gain=10
  MATLAB Function : MATLAB Function  TreatAsAtomicUnit=on
  MATLAB Function1 : MATLAB Function  TreatAsAtomicUnit=on
  MATLAB Function14 : MATLAB Function  TreatAsAtomicUnit=on
  Mux{,1..3} (4 alike) : Mux
  Product{,1..3} (4 alike) : Product  Inputs=3
  Product4 : Product
  Product5 : Product
  Product6 : Product
  Saturation : Saturate  UpperLimit=2500  LowerLimit=0
  Saturation1 : Saturate  UpperLimit=0  LowerLimit=-1000
  Sign : Signum
  Switch : Switch  Criteria=u2 > Threshold
  Switch1 : Switch  Criteria=u2 > Threshold
  Switch2 : Switch  Criteria=u2 > Threshold
  Torque_NegLimitRegene : Outport
  Torque_Normal : Outport  Port=2
  wires:
  torque/1 -> MATLAB Function14/1(Throttle), MATLAB Function/1(Throttle), Divide/2
  Sign/1 -> [target_velocity], Divide/1
  Divide/1 -> Product4/1, Gain2/1
  T_max/1 -> Gain1/1
  MATLAB Function/1(factor_F) -> [factor_F]
  1-D Lookup Table5/1 -> [factor_R]
  1-D Lookup Table4/1 -> [factor_L]
  steer/1 -> 1-D Lookup Table5/1, 1-D Lookup Table4/1
  Gain1/1 -> [T_max]
  [factor_F] -> Product/2
  [factor_R] -> Product/3
  [Torque] -> Product/1
  [factor_F] -> Product1/2
  [factor_L] -> Product1/3
  [Torque] -> Product1/1
  [Torque] -> Product2/1
  [factor_R] -> Product2/2
  [Torque] -> Product3/1
  [factor_L] -> Product3/2
  Product4/1 -> [Torque]
  [T_max] -> Product4/2
  Mux/1 -> Saturation/1
  MATLAB Function14/1(factor_R) -> [factor_Rear]
  [factor_Rear] -> Product2/3
  [factor_Rear] -> Product3/3
  Product/1 -> Mux/2
  Product1/1 -> Mux/1
  Product3/1 -> Mux/3
  Product2/1 -> Mux/4
  Saturation/1 -> Product5/2
  target_velocity/1 -> Sign/1
  [target_velocity] -> Product5/1
  [target_velocity] -> Gain/1
  Gain/1 -> Product6/1
  Saturation1/1 -> Product6/2
  Gain2/1 -> Saturation1/1
  reset_state/1 -> [reset_state]
  [reset_state] -> Switch/2
  Switch/1 -> Torque_NegLimitRegene/1
  Constant/1 -> Mux1/3, Mux1/4, Mux1/2, Mux1/1
  Mux1/1 -> [torque_zero]
  [reset_state] -> Switch1/2
  Product5/1 -> Switch1/3
  [torque_zero] -> Switch1/1
  Switch1/1 -> Torque_Normal/1
  flag_regen/1 -> Switch2/2
  Switch2/1 -> Switch/3
  SOC/1 -> MATLAB Function1/1(SOC)
  [torque_regen] -> Switch2/1
  AMKSpeed/1 -> MATLAB Function1/4(AMKSpeed)
  MaxCellVolt/1 -> MATLAB Function1/5(MaxCellVolt)
  brake_pressure_f/1 -> MATLAB Function1/2(brake_pressure_f)
  brake_pressure_r/1 -> MATLAB Function1/3(brake_pressure_r)
  [torque_zero] -> Switch/1
  MATLAB Function1/1(torque_regen_f) -> Mux2/2, Mux2/1
  MATLAB Function1/2(torque_regen_r) -> Mux2/3, Mux2/4
  Mux2/1 -> [torque_regen]
  Product6/1 -> Mux3/4, Mux3/3, Mux3/1, Mux3/2
  Mux3/1 -> [torque_reverse]
  [torque_reverse] -> Switch2/3

== system E55_1030/Function-Call Subsystem2/If Action Subsystem16 ==
  Action Port : ActionPort  ActionPortLabel=else
  Constant2 : Constant
  DeratingRatio : Outport
  wires:
  Constant2/1 -> DeratingRatio/1

== system E55_1030/Function-Call Subsystem2/If Action Subsystem20 ==
  Action Port : ActionPort  ActionPortLabel=elseif(u2 == 3)
  Bus Creator : BusCreator  Inputs=4
  DcOn : Constant
  Enable : Constant
  ErrorReset : Constant  Value=0
  InverterOn : Constant
  ready_to_go : Outport
  wires:
  InverterOn/1 -> Bus Creator/2  "InverterOn"
  DcOn/1 -> Bus Creator/1  "DcOn"
  Enable/1 -> Bus Creator/3  "Enable"
  Bus Creator/1 -> ready_to_go/1
  ErrorReset/1 -> Bus Creator/4  "ErrorReset"

== system E55_1030/Function-Call Subsystem2/If Action Subsystem21 ==
  Action Port : ActionPort  ActionPortLabel=else
  Bus Creator : BusCreator  Inputs=4
  DcOn : Constant  Value=0
  Enable : Constant  Value=0
  ErrorReset : Constant  Value=0
  InverterOn : Constant  Value=0
  standby : Outport
  wires:
  InverterOn/1 -> Bus Creator/2  "InverterOn"
  DcOn/1 -> Bus Creator/1  "DcOn"
  Enable/1 -> Bus Creator/3  "Enable"
  Bus Creator/1 -> standby/1
  ErrorReset/1 -> Bus Creator/4  "ErrorReset"

== system E55_1030/Function-Call Subsystem2/If Action Subsystem22 ==
  Action Port : ActionPort  ActionPortLabel=if(u1 > 0)
  Bus Creator : BusCreator  Inputs=4
  DcOn : Constant  Value=0
  Enable : Constant  Value=0
  ErrorReset : Constant
  InverterOn : Constant  Value=0
  Reset : Outport
  wires:
  DcOn/1 -> Bus Creator/1  "DcOn"
  InverterOn/1 -> Bus Creator/2  "InverterOn"
  Enable/1 -> Bus Creator/3  "Enable"
  ErrorReset/1 -> Bus Creator/4  "ErrorReset"
  Bus Creator/1 -> Reset/1

== system E55_1030/Function-Call Subsystem2/If Action Subsystem5 ==
  In1 : Inport
  Action Port : ActionPort  ActionPortLabel=if(u1<6.66)
  1-D Lookup Table : Lookup_n-D  NumberOfTableDimensions=1  BreakpointsForDimension1=linspace(0,6.66,473)  Table=SOC_Discharge  InternalRulePriority=Speed  RndMeth=Simplest  InputSameDT=on
  Constant : Constant  Value=400
  Divide : Product  Inputs=*/
  DeratingRatio : Outport
  wires:
  In1/1 -> 1-D Lookup Table/1
  1-D Lookup Table/1 -> Divide/1
  Constant/1 -> Divide/2
  Divide/1 -> DeratingRatio/1

== system E55_1030/Function-Call Subsystem2/If Action Subsystem7 ==
  Action Port : ActionPort  ActionPortLabel=if(u1 > 1)
  Constant15 : Constant  Value=255  OutDataTypeStr=uint8
  Out1 : Outport
  wires:
  Constant15/1 -> Out1/1

== system E55_1030/Function-Call Subsystem2/If Action Subsystem9 ==
  Action Port : ActionPort  ActionPortLabel=else
  Constant15 : Constant  Value=0  OutDataTypeStr=uint8
  Out1 : Outport
  wires:
  Constant15/1 -> Out1/1

== system E55_1030/Function-Call Subsystem2/SMC ==
  yaw_rate : Inport
  yaw_rate_d : Inport  Port=2
  side_slip_angle : Inport  Port=3
  side_slip_angle_d : Inport  Port=4
  Abs : Abs
  Abs1 : Abs
  Constant : Constant  Value=Iz
  Discrete Derivative : simulink/Discrete/Discrete Derivative  gainval=1.0  ICPrevScaledInput=0.0  OutMin=[]  OutMax=[]  OutDataType=fixdt(1, 16)  OutScaling=2^-10  DoSatur=off
  Discrete-Time Integrator : DiscreteIntegrator  SampleTime=-1  ICPrevOutput=DiscIntNeverNeededParam  ICPrevScaledInput=DiscIntNeverNeededParam
  Gain : Gain  Gain=xi
  Gain1 : Gain  Gain=1/1
  Gain2 : Gain  Gain=xi
  Product : Product
  Saturation : Saturate  UpperLimit=150  LowerLimit=-150
  Sign : Signum
  Subtract{,1,3..4} (4 alike) : Sum  Inputs=+-
  Subtract2 : Sum
  Subtract5 : Sum  Inputs=--+
  Subtract6 : Sum  Inputs=-+
  Switch : Switch  Criteria=u2 > Threshold  Threshold=1
  k : Gain  Gain=0.3
  ki : Gain  Gain=2
  ε : Gain  Gain=0.01
  ΔMz : Outport
  wires:
  Gain2/1 -> Subtract4/2
  Subtract5/1 -> Product/2
  ε/1 -> Subtract5/2
  Subtract4/1 -> Discrete Derivative/1
  Discrete-Time Integrator/1 -> ki/1
  k/1 -> Subtract5/1
  Subtract3/1 -> Gain2/1
  Constant/1 -> Product/1
  Sign/1 -> Switch/1
  Subtract2/1 -> Gain1/1, Discrete-Time Integrator/1, k/1, Sign/1, Abs/1  "S"
  ki/1 -> Subtract6/1
  Subtract1/1 -> Gain/1
  yaw_rate_d/1 -> Subtract4/1, Subtract/2
  Gain/1 -> Subtract2/2
  yaw_rate/1 -> Subtract/1
  side_slip_angle_d/1 -> Subtract3/2, Subtract1/2
  Subtract/1 -> Subtract2/1
  side_slip_angle/1 -> Subtract3/1, Subtract1/1
  Abs/1 -> Switch/2
  Gain1/1 -> Switch/3
  Product/1 -> Subtract6/2
  Switch/1 -> ε/1
  Saturation/1 -> Abs1/1  "ΔMz"
  Subtract6/1 -> Saturation/1
  Discrete Derivative/1 -> Subtract5/3
  Abs1/1 -> ΔMz/1

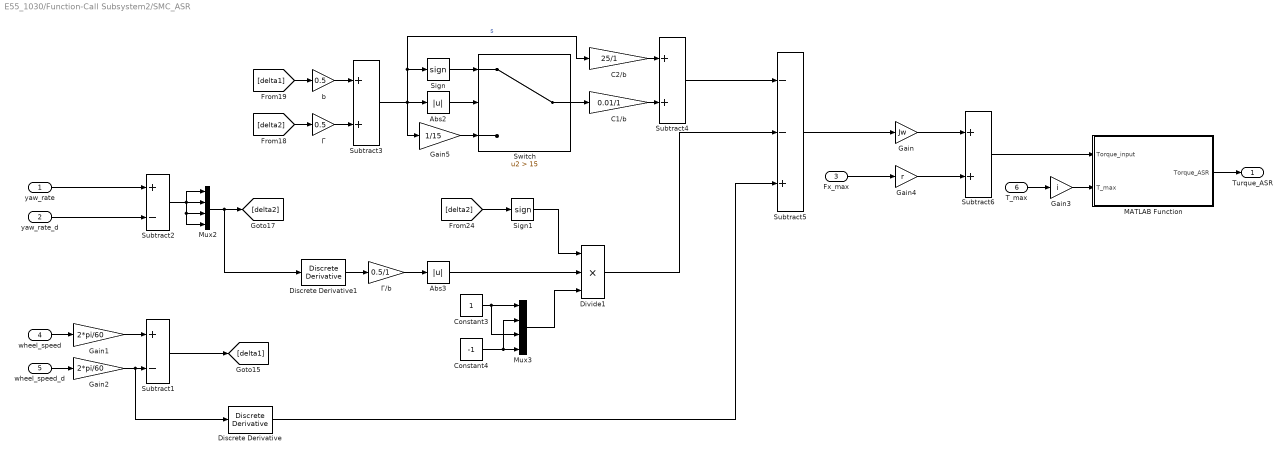
== system E55_1030/Function-Call Subsystem2/SMC_ASR ==
  yaw_rate : Inport
  yaw_rate_d : Inport  Port=2
  Fx_max : Inport  Port=3
  wheel_speed : Inport  Port=4
  wheel_speed_d : Inport  Port=5
  T_max : Inport  Port=6
  Abs2 : Abs
  Abs3 : Abs
  C1/b : Gain  Gain=0.01/1
  C2/b : Gain  Gain=25/1
  Constant3 : Constant
  Constant4 : Constant  Value=-1
  Discrete Derivative : simulink/Discrete/Discrete Derivative  gainval=1.0  ICPrevScaledInput=0.0  OutMin=[]  OutMax=[]  OutDataType=fixdt(1, 16)  OutScaling=2^-10  DoSatur=off
  Discrete Derivative1 : simulink/Discrete/Discrete Derivative  gainval=1.0  ICPrevScaledInput=0.0  OutMin=[]  OutMax=[]  OutDataType=fixdt(1, 16)  OutScaling=2^-10  DoSatur=off
  Divide1 : Product  Inputs=***
  Gain : Gain  Gain=Jw
  Gain1 : Gain  Gain=2*pi/60
  Gain2 : Gain  Gain=2*pi/60
  Gain3 : Gain  Gain=i
  Gain4 : Gain  Gain=r
  Gain5 : Gain  Gain=1/15
  MATLAB Function : MATLAB Function  TreatAsAtomicUnit=on
  Mux2 : Mux
  Mux3 : Mux
  Sign : Signum
  Sign1 : Signum
  Subtract1 : Sum  Inputs=+-
  Subtract2 : Sum  Inputs=+-
  Subtract3 : Sum
  Subtract4 : Sum
  Subtract5 : Sum  Inputs=--+
  Subtract6 : Sum
  Switch : Switch  Criteria=u2 > Threshold  Threshold=15
  b : Gain  Gain=0.5
  Г : Gain  Gain=0.5
  Г/b : Gain  Gain=0.5/1
  Turque_ASR : Outport
  wires:
  Constant4/1 -> Mux3/2, Mux3/4
  Gain5/1 -> Switch/3
  wheel_speed_d/1 -> Gain2/1
  b/1 -> Subtract3/1
  Subtract3/1 -> Gain5/1, Sign/1, C2/b/1, Abs2/1  "s"
  Subtract2/1 -> Mux2/1, Mux2/4, Mux2/3, Mux2/2
  [delta1] -> b/1
  Constant3/1 -> Mux3/3, Mux3/1
  Discrete Derivative/1 -> Subtract5/3
  Г/1 -> Subtract3/2
  Subtract5/1 -> Gain/1
  yaw_rate/1 -> Subtract2/1
  Divide1/1 -> Subtract5/2
  Gain/1 -> Subtract6/1
  Г/b/1 -> Abs3/1
  Discrete Derivative1/1 -> Г/b/1
  Subtract1/1 -> [delta1]
  Abs2/1 -> Switch/2
  Switch/1 -> C1/b/1
  C1/b/1 -> Subtract4/2
  Gain2/1 -> Discrete Derivative/1, Subtract1/2
  Subtract4/1 -> Subtract5/1
  Mux2/1 -> Discrete Derivative1/1, [delta2]
  Sign/1 -> Switch/1
  C2/b/1 -> Subtract4/1
  Mux3/1 -> Divide1/3
  [delta2] -> Г/1
  [delta2] -> Sign1/1
  Abs3/1 -> Divide1/2
  Sign1/1 -> Divide1/1
  yaw_rate_d/1 -> Subtract2/2
  wheel_speed/1 -> Gain1/1
  Fx_max/1 -> Gain4/1
  Gain1/1 -> Subtract1/1
  Gain4/1 -> Subtract6/2
  MATLAB Function/1(Torque_ASR) -> Turque_ASR/1
  Subtract6/1 -> MATLAB Function/1(Torque_input)
  T_max/1 -> Gain3/1
  Gain3/1 -> MATLAB Function/2(T_max)

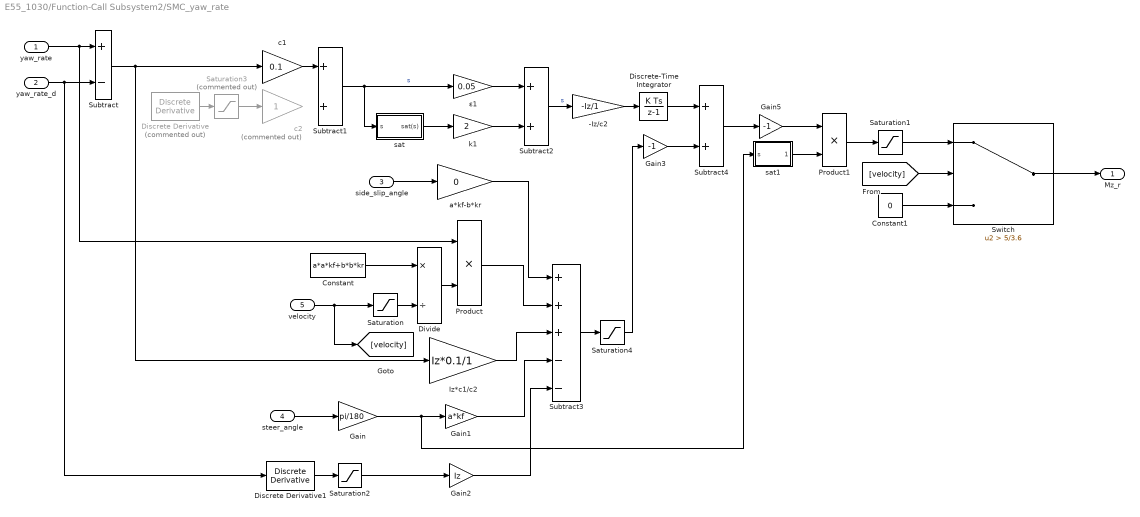
== system E55_1030/Function-Call Subsystem2/SMC_yaw_rate ==
  yaw_rate : Inport
  yaw_rate_d : Inport  Port=2
  side_slip_angle : Inport  Port=3
  steer_angle : Inport  Port=4
  velocity : Inport  Port=5
  -Iz/c2 : Gain  Gain=-Iz/1
  Constant : Constant  Value=a*a*kf+b*b*kr
  Constant1 : Constant  Value=0
  Discrete Derivative : simulink/Discrete/Discrete Derivative  Commented=on  gainval=1.0  ICPrevScaledInput=0.0  OutMin=[]  OutMax=[]  OutDataType=fixdt(1, 16)  OutScaling=2^-10  DoSatur=off
  Discrete Derivative1 : simulink/Discrete/Discrete Derivative  gainval=1.0  ICPrevScaledInput=0.0  OutMin=[]  OutMax=[]  OutDataType=fixdt(1, 16)  OutScaling=2^-10  DoSatur=off
  Discrete-Time Integrator : DiscreteIntegrator  SampleTime=-1  ICPrevOutput=DiscIntNeverNeededParam  ICPrevScaledInput=DiscIntNeverNeededParam
  Divide : Product  Inputs=*/
  Gain : Gain  Gain=pi/180
  Gain1 : Gain  Gain=a*kf
  Gain2 : Gain  Gain=Iz
  Gain3 : Gain  Gain=-1
  Gain5 : Gain  Gain=-1
  Iz*c1/c2 : Gain  Gain=Iz*0.1/1
  Product : Product
  Product1 : Product
  Saturation : Saturate  UpperLimit=Inf  LowerLimit=5/3.6
  Saturation1 : Saturate  UpperLimit=300  LowerLimit=-300
  Saturation2 : Saturate  UpperLimit=5  LowerLimit=-5
  Saturation3 : Saturate  Commented=on  UpperLimit=5  LowerLimit=-5
  Saturation4 : Saturate  UpperLimit=1000  LowerLimit=-1000
  Subtract : Sum  Inputs=+-
  Subtract1 : Sum
  Subtract2 : Sum
  Subtract3 : Sum  Inputs=+++--
  Subtract4 : Sum
  Switch : Switch  Criteria=u2 > Threshold  Threshold=5/3.6
  a*kf-b*kr : Gain  Gain=0
  c1 : Gain  Gain=0.1
  c2 : Gain  Commented=on
  k1 : Gain  Gain=2
  sat : Subsystem
  sat1 : Subsystem
  ε1 : Gain  Gain=0.05
  Mz_r : Outport
  wires:
  yaw_rate/1 -> Product/1, Subtract/1
  Subtract/1 -> c1/1, Iz*c1/c2/1
  Discrete Derivative/1 -> Saturation3/1
  c1/1 -> Subtract1/1
  Subtract1/1 -> sat/1(s), ε1/1  "s"
  sat/1(sat(s)) -> k1/1
  ε1/1 -> Subtract2/1
  k1/1 -> Subtract2/2
  Subtract2/1 -> -Iz/c2/1  "s"
  -Iz/c2/1 -> Discrete-Time Integrator/1
  side_slip_angle/1 -> a*kf-b*kr/1
  Discrete Derivative1/1 -> Saturation2/1
  Constant/1 -> Divide/1
  Divide/1 -> Product/2
  a*kf-b*kr/1 -> Subtract3/1
  Product/1 -> Subtract3/2
  Iz*c1/c2/1 -> Subtract3/3
  Gain1/1 -> Subtract3/4
  Gain2/1 -> Subtract3/5
  Subtract3/1 -> Saturation4/1
  Subtract4/1 -> Gain5/1
  Saturation/1 -> Divide/2
  velocity/1 -> [velocity], Saturation/1
  yaw_rate_d/1 -> Discrete Derivative1/1, Subtract/2
  Saturation2/1 -> Gain2/1
  Product1/1 -> Saturation1/1
  sat1/1(sat(s)) -> Product1/2
  Gain5/1 -> Product1/1
  steer_angle/1 -> Gain/1
  Saturation3/1 -> c2/1
  Gain/1 -> sat1/1(s), Gain1/1
  Saturation4/1 -> Gain3/1
  Discrete-Time Integrator/1 -> Subtract4/1
  Gain3/1 -> Subtract4/2
  [velocity] -> Switch/2
  Saturation1/1 -> Switch/1
  Constant1/1 -> Switch/3
  Switch/1 -> Mz_r/1

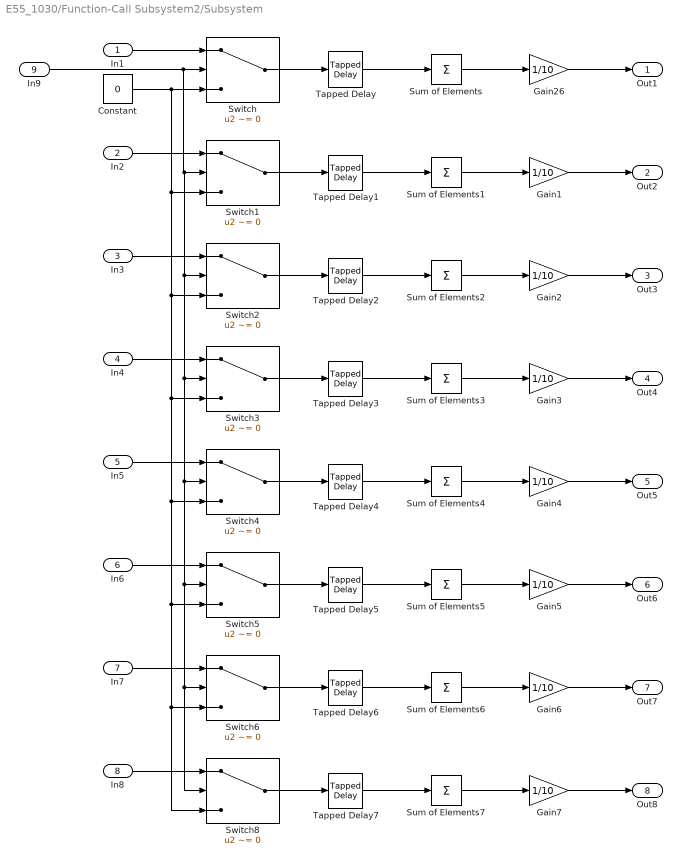
== system E55_1030/Function-Call Subsystem2/Subsystem ==
  In1 : Inport
  In2 : Inport  Port=2
  In3 : Inport  Port=3
  In4 : Inport  Port=4
  In5 : Inport  Port=5
  In6 : Inport  Port=6
  In7 : Inport  Port=7
  In8 : Inport  Port=8
  In9 : Inport  Port=9
  Constant : Constant  Value=0
  Gain{1..7,26} (8 alike) : Gain  Gain=1/10
  Sum of Elements{,1..7} (8 alike) : Sum  Inputs=+
  Switch{,1..6,8} (8 alike) : Switch  Criteria=u2 ~= 0
  Tapped Delay{,1..7} (8 alike) : simulink/Discrete/Tapped Delay  vinit=0.0  samptime=-1  NumDelays=10  DelayOrder=Oldest  includeCurrent=off
  Out1 : Outport
  Out2 : Outport  Port=2
  Out3 : Outport  Port=3
  Out4 : Outport  Port=4
  Out5 : Outport  Port=5
  Out6 : Outport  Port=6
  Out7 : Outport  Port=7
  Out8 : Outport  Port=8
  wires:
  Gain26/1 -> Out1/1
  Tapped Delay/1 -> Sum of Elements/1
  Sum of Elements/1 -> Gain26/1
  Switch/1 -> Tapped Delay/1
  In1/1 -> Switch/1
  In9/1 -> Switch4/2, Switch8/2, Switch6/2, Switch5/2, Switch3/2, Switch2/2, Switch1/2, Switch/2
  Constant/1 -> Switch5/3, Switch8/3, Switch6/3, Switch4/3, Switch3/3, Switch2/3, Switch1/3, Switch/3
  In2/1 -> Switch1/1
  In3/1 -> Switch2/1
  In4/1 -> Switch3/1
  In5/1 -> Switch4/1
  In6/1 -> Switch5/1
  In7/1 -> Switch6/1
  In8/1 -> Switch8/1
  Switch1/1 -> Tapped Delay1/1
  Gain1/1 -> Out2/1
  Switch2/1 -> Tapped Delay2/1
  Gain2/1 -> Out3/1
  Switch3/1 -> Tapped Delay3/1
  Gain3/1 -> Out4/1
  Switch4/1 -> Tapped Delay4/1
  Gain4/1 -> Out5/1
  Switch5/1 -> Tapped Delay5/1
  Gain5/1 -> Out6/1
  Switch6/1 -> Tapped Delay6/1
  Gain6/1 -> Out7/1
  Switch8/1 -> Tapped Delay7/1
  Gain7/1 -> Out8/1
  Sum of Elements1/1 -> Gain1/1
  Tapped Delay1/1 -> Sum of Elements1/1
  Tapped Delay2/1 -> Sum of Elements2/1
  Sum of Elements2/1 -> Gain2/1
  Sum of Elements3/1 -> Gain3/1
  Tapped Delay3/1 -> Sum of Elements3/1
  Tapped Delay4/1 -> Sum of Elements4/1
  Sum of Elements4/1 -> Gain4/1
  Sum of Elements5/1 -> Gain5/1
  Tapped Delay5/1 -> Sum of Elements5/1
  Tapped Delay6/1 -> Sum of Elements6/1
  Sum of Elements6/1 -> Gain6/1
  Sum of Elements7/1 -> Gain7/1
  Tapped Delay7/1 -> Sum of Elements7/1

== system E55_1030/Function-Call Subsystem2/Subsystem1 ==
  CAN_OK : Inport
  CAN ID : Inport  Port=2
  CAN Msg : Inport  Port=3
  function : TriggerPort  TriggerType=function-call  VariantControl=(inherit)
  Bus Creator : BusCreator  Inputs=4
  Enabled Subsystem : Subsystem  TreatAsAtomicUnit=on
  284_data : Outport
  wires:
  CAN_OK/1 -> Enabled Subsystem/Enable
  CAN ID/1 -> Enabled Subsystem/1(In1)
  CAN Msg/1 -> Enabled Subsystem/2(In2)
  Enabled Subsystem/2(284_Error) -> Bus Creator/2  "bError"
  Enabled Subsystem/1(284_ActualVelocity) -> Bus Creator/1  "AMK_Speed"
  Bus Creator/1 -> 284_data/1
  Enabled Subsystem/3(284_Id) -> Bus Creator/3  "Id"
  Enabled Subsystem/4(284_Iq) -> Bus Creator/4  "Iq"

== system E55_1030/Function-Call Subsystem2/Subsystem10 ==
  CAN_OK : Inport
  CAN ID : Inport  Port=2
  CAN Msg : Inport  Port=3
  function : TriggerPort  TriggerType=function-call  VariantControl=(inherit)
  Bus Creator : BusCreator  Inputs=5
  Enabled Subsystem : Subsystem  TreatAsAtomicUnit=on
  BMS_data : Outport
  wires:
  CAN_OK/1 -> Enabled Subsystem/Enable  "CAN_OK"
  CAN ID/1 -> Enabled Subsystem/1(In1)
  CAN Msg/1 -> Enabled Subsystem/2(In2)
  Bus Creator/1 -> BMS_data/1
  Enabled Subsystem/1(BMSState) -> Bus Creator/1  "BMSState"
  Enabled Subsystem/2(CellTemp) -> Bus Creator/2  "CellTemp"
  Enabled Subsystem/3(MaxCellVolt) -> Bus Creator/3  "MaxCellVolt"
  Enabled Subsystem/4(MinCellVolt) -> Bus Creator/4  "MinCellVolt"
  Enabled Subsystem/5(SOC) -> Bus Creator/5  "SOC"
